simulink model "lab06_02_sat"  (R2018b)
settings: Solver=VariableStepAuto  StartTime=0.0  StopTime=10.0  FixedStep=0.00001  RelTol=1e-3
libraries: simulink x1
settings Model: Creator=Еня  LastModifiedBy=Еня

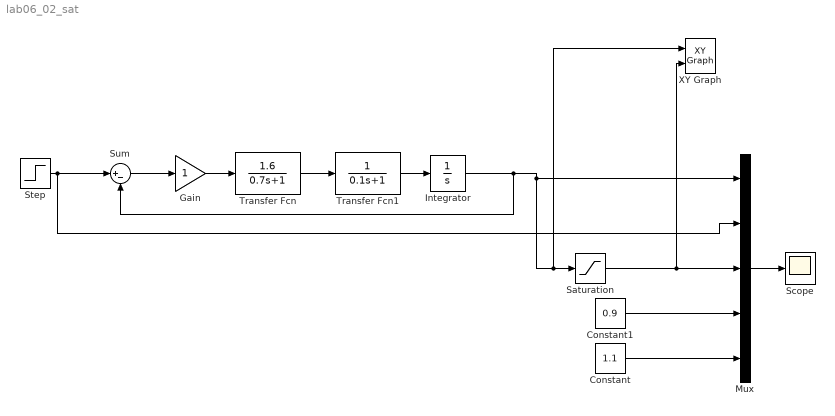
== system lab06_02_sat ==
  Constant : Constant  Value=1.1
  Constant1 : Constant  Value=0.9
  Gain : Gain
  Integrator : Integrator
  Mux : Mux  Inputs=5
  Saturation : Saturate  UpperLimit=1.1  LowerLimit=0.9
  Scope : Scope
  Step : Step  Time=0  SampleTime=0
  Sum : Sum  Inputs=|+-
  Transfer Fcn : TransferFcn  Numerator=[1.6]  Denominator=[0.7 1]
  Transfer Fcn1 : TransferFcn  Denominator=[0.1 1]
  XY Graph : simulink/Sinks/XY Graph  xmin=0  xmax=1.5  ymin=0  ymax=1.5  st=-1
  wires:
  Step/1 -> Mux/2, Sum/1
  Sum/1 -> Gain/1
  Gain/1 -> Transfer Fcn/1
  Transfer Fcn/1 -> Transfer Fcn1/1
  Transfer Fcn1/1 -> Integrator/1
  Mux/1 -> Scope/1
  Integrator/1 -> Saturation/1, XY Graph/1, Mux/1, Sum/2
  Saturation/1 -> Mux/3, XY Graph/2
  Constant1/1 -> Mux/4
  Constant/1 -> Mux/5
